simulink model "L400_airframe"  (R2024b)
settings: Solver=FixedStepAuto  StartTime=0  StopTime=10  FixedStep=5/1000  RelTol=1e-3
values from neighbouring files (symbols this model uses):
  db =     [L400_airframe_data.mat]
undefined symbols (not defined in the file or in its folder): lambda
libraries: aerolibconvert2 x16, simulink x6, matrix_library x4, aerolibactuator x2, shared6dof x1, aerolibtransform2 x1
(part 3 of 4)

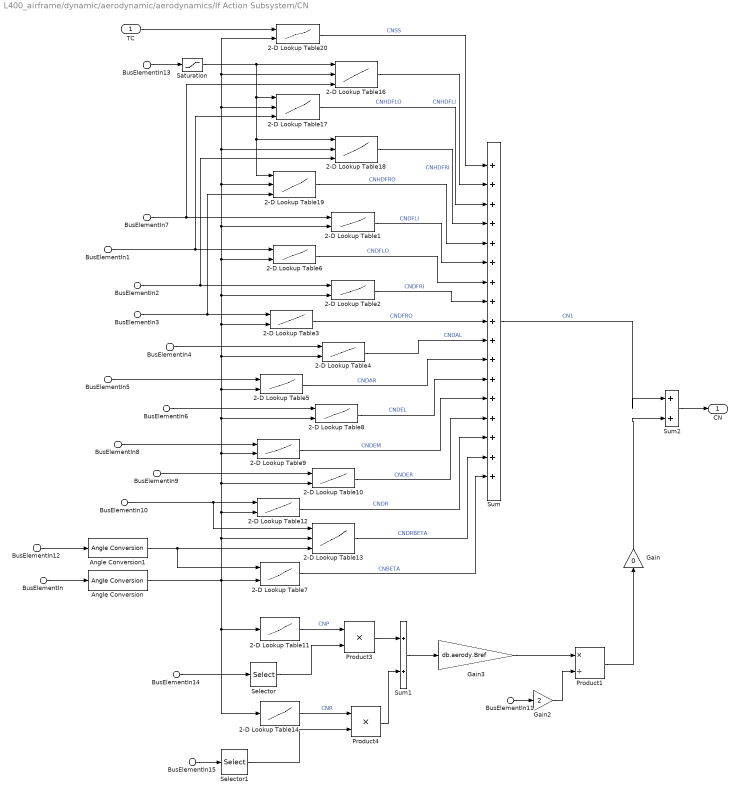
== system L400_airframe/dynamic/aerodynamic/aerodynamics/If Action Subsystem/CN ==
  TC : Inport
  BusElementIn7 : Inport  Port=2  PortName=surface  Element=DFLI
  BusElementIn1 : Inport  Port=2  PortName=surface  Element=DFLO
  BusElementIn2 : Inport  Port=2  PortName=surface  Element=DFRI
  BusElementIn3 : Inport  Port=2  PortName=surface  Element=DFRO
  BusElementIn4 : Inport  Port=2  PortName=surface  Element=DAL
  BusElementIn5 : Inport  Port=2  PortName=surface  Element=DAR
  BusElementIn6 : Inport  Port=2  PortName=surface  Element=DEL
  BusElementIn8 : Inport  Port=2  PortName=surface  Element=DEM
  BusElementIn9 : Inport  Port=2  PortName=surface  Element=DER
  BusElementIn10 : Inport  Port=2  PortName=surface  Element=DR
  BusElementIn : Inport  Port=3  PortName=state  Element=aircraft.airdata.alpha
  BusElementIn12 : Inport  Port=3  PortName=state  Element=aircraft.airdata.beta
  BusElementIn11 : Inport  Port=3  PortName=state  Element=aircraft.airdata.airspeed
  BusElementIn13 : Inport  Port=3  PortName=state  Element=aircraft.position.agl
  BusElementIn14 : Inport  Port=3  PortName=state  Element=aircraft.attitude.p_q_r
  BusElementIn15 : Inport  Port=3  PortName=state  Element=aircraft.attitude.p_q_r
  2-D Lookup Table1 : Lookup_n-D  LookupTableObject=''  BreakpointsForDimension1=db.aerody.VDF  BreakpointsForDimension2=db.aerody.VALPHA  BreakpointsForDimension1FirstPoint=10  BreakpointsForDimension2FirstPoint=10  BreakpointsForDimension1Spacing=12  BreakpointsForDimension2Spacing=12  IndexSearchMethod=Linear search  BeginIndexSearchUsingPreviousIndexResult=on  Table=db.aerody.CNDFLI  ExtrapMethod=Clip  DiagnosticForOutOfRangeInput=Warning  InternalRulePriority=Speed  RndMeth=Simplest
      settings: InputPortMap=u0,u1
  2-D Lookup Table10 : Lookup_n-D  LookupTableObject=''  BreakpointsForDimension1=db.aerody.VDE  BreakpointsForDimension2=db.aerody.VALPHA  BreakpointsForDimension1FirstPoint=10  BreakpointsForDimension2FirstPoint=10  BreakpointsForDimension1Spacing=12  BreakpointsForDimension2Spacing=12  IndexSearchMethod=Linear search  BeginIndexSearchUsingPreviousIndexResult=on  Table=db.aerody.CNDER  ExtrapMethod=Clip  DiagnosticForOutOfRangeInput=Warning  InternalRulePriority=Speed  RndMeth=Simplest
      settings: InputPortMap=u0,u1
  2-D Lookup Table11 : Lookup_n-D  NumberOfTableDimensions=1  LookupTableObject=''  BreakpointsForDimension1=db.dds.VALPHA  BreakpointsForDimension2=db.aerody.VALPHA  BreakpointsForDimension1FirstPoint=10  BreakpointsForDimension2FirstPoint=10  BreakpointsForDimension1Spacing=12  BreakpointsForDimension2Spacing=12  IndexSearchMethod=Linear search  BeginIndexSearchUsingPreviousIndexResult=on  Table=db.dds.CNP  ExtrapMethod=Clip  DiagnosticForOutOfRangeInput=Warning  InternalRulePriority=Speed  RndMeth=Simplest
  2-D Lookup Table12 : Lookup_n-D  LookupTableObject=''  BreakpointsForDimension1=db.aerody.VDR  BreakpointsForDimension2=db.aerody.VALPHA  BreakpointsForDimension1FirstPoint=10  BreakpointsForDimension2FirstPoint=10  BreakpointsForDimension1Spacing=12  BreakpointsForDimension2Spacing=12  IndexSearchMethod=Linear search  BeginIndexSearchUsingPreviousIndexResult=on  Table=db.aerody.CNDR  ExtrapMethod=Clip  DiagnosticForOutOfRangeInput=Warning  InternalRulePriority=Speed  RndMeth=Simplest
      settings: InputPortMap=u0,u1
  2-D Lookup Table13 : Lookup_n-D  NumberOfTableDimensions=3  LookupTableObject=''  BreakpointsForDimension1=db.aerody.VDR  BreakpointsForDimension2=db.aerody.VALPHA  BreakpointsForDimension3=db.aerody.VBETA  BreakpointsForDimension1FirstPoint=10  BreakpointsForDimension2FirstPoint=10  BreakpointsForDimension1Spacing=12  BreakpointsForDimension2Spacing=12  IndexSearchMethod=Linear search  BeginIndexSearchUsingPreviousIndexResult=on  Table=db.aerody.CNDRBETA  ExtrapMethod=Clip  DiagnosticForOutOfRangeInput=Warning  InternalRulePriority=Speed  RndMeth=Simplest
      settings: InputPortMap=u0,u1,u2
  2-D Lookup Table14 : Lookup_n-D  NumberOfTableDimensions=1  LookupTableObject=''  BreakpointsForDimension1=db.dds.VALPHA  BreakpointsForDimension2=db.aerody.VALPHA  BreakpointsForDimension1FirstPoint=10  BreakpointsForDimension2FirstPoint=10  BreakpointsForDimension1Spacing=12  BreakpointsForDimension2Spacing=12  IndexSearchMethod=Linear search  BeginIndexSearchUsingPreviousIndexResult=on  Table=db.dds.CNR  ExtrapMethod=Clip  DiagnosticForOutOfRangeInput=Warning  InternalRulePriority=Speed  RndMeth=Simplest
  2-D Lookup Table16 : Lookup_n-D  NumberOfTableDimensions=3  LookupTableObject=''  BreakpointsForDimension1=db.aerody.VH  BreakpointsForDimension2=db.aerody.VALPHA  BreakpointsForDimension3=db.aerody.VDF  BreakpointsForDimension1FirstPoint=10  BreakpointsForDimension2FirstPoint=10  BreakpointsForDimension1Spacing=12  BreakpointsForDimension2Spacing=12  IndexSearchMethod=Linear search  BeginIndexSearchUsingPreviousIndexResult=on  Table=db.aerody.CNHDFLI  ExtrapMethod=Clip  DiagnosticForOutOfRangeInput=Warning  InternalRulePriority=Speed  RndMeth=Simplest
      settings: InputPortMap=u0,u1,u2
  2-D Lookup Table17 : Lookup_n-D  NumberOfTableDimensions=3  LookupTableObject=''  BreakpointsForDimension1=db.aerody.VH  BreakpointsForDimension2=db.aerody.VALPHA  BreakpointsForDimension3=db.aerody.VDF  BreakpointsForDimension1FirstPoint=10  BreakpointsForDimension2FirstPoint=10  BreakpointsForDimension1Spacing=12  BreakpointsForDimension2Spacing=12  IndexSearchMethod=Linear search  BeginIndexSearchUsingPreviousIndexResult=on  Table=db.aerody.CNHDFLO  ExtrapMethod=Clip  DiagnosticForOutOfRangeInput=Warning  InternalRulePriority=Speed  RndMeth=Simplest
      settings: InputPortMap=u0,u1,u2
  2-D Lookup Table18 : Lookup_n-D  NumberOfTableDimensions=3  LookupTableObject=''  BreakpointsForDimension1=db.aerody.VH  BreakpointsForDimension2=db.aerody.VALPHA  BreakpointsForDimension3=db.aerody.VDF  BreakpointsForDimension1FirstPoint=10  BreakpointsForDimension2FirstPoint=10  BreakpointsForDimension1Spacing=12  BreakpointsForDimension2Spacing=12  IndexSearchMethod=Linear search  BeginIndexSearchUsingPreviousIndexResult=on  Table=db.aerody.CNHDFRI  ExtrapMethod=Clip  DiagnosticForOutOfRangeInput=Warning  InternalRulePriority=Speed  RndMeth=Simplest
      settings: InputPortMap=u0,u1,u2
  2-D Lookup Table19 : Lookup_n-D  NumberOfTableDimensions=3  LookupTableObject=''  BreakpointsForDimension1=db.aerody.VH  BreakpointsForDimension2=db.aerody.VALPHA  BreakpointsForDimension3=db.aerody.VDF  BreakpointsForDimension1FirstPoint=10  BreakpointsForDimension2FirstPoint=10  BreakpointsForDimension1Spacing=12  BreakpointsForDimension2Spacing=12  IndexSearchMethod=Linear search  BeginIndexSearchUsingPreviousIndexResult=on  Table=db.aerody.CNHDFRO  ExtrapMethod=Clip  DiagnosticForOutOfRangeInput=Warning  InternalRulePriority=Speed  RndMeth=Simplest
      settings: InputPortMap=u0,u1,u2
  2-D Lookup Table2 : Lookup_n-D  LookupTableObject=''  BreakpointsForDimension1=db.aerody.VDF  BreakpointsForDimension2=db.aerody.VALPHA  BreakpointsForDimension1FirstPoint=10  BreakpointsForDimension2FirstPoint=10  BreakpointsForDimension1Spacing=12  BreakpointsForDimension2Spacing=12  IndexSearchMethod=Linear search  BeginIndexSearchUsingPreviousIndexResult=on  Table=db.aerody.CNDFRI  ExtrapMethod=Clip  DiagnosticForOutOfRangeInput=Warning  InternalRulePriority=Speed  RndMeth=Simplest
      settings: InputPortMap=u0,u1
  2-D Lookup Table20 : Lookup_n-D  LookupTableObject=''  BreakpointsForDimension1=db.aerody.VTC  BreakpointsForDimension2=db.aerody.VALPHA  BreakpointsForDimension1FirstPoint=10  BreakpointsForDimension2FirstPoint=10  BreakpointsForDimension1Spacing=12  BreakpointsForDimension2Spacing=12  IndexSearchMethod=Linear search  BeginIndexSearchUsingPreviousIndexResult=on  Table=db.aerody.CNSS  ExtrapMethod=Clip  DiagnosticForOutOfRangeInput=Warning  InternalRulePriority=Speed  RndMeth=Simplest
      settings: InputPortMap=u0,u1
  2-D Lookup Table3 : Lookup_n-D  LookupTableObject=''  BreakpointsForDimension1=db.aerody.VDF  BreakpointsForDimension2=db.aerody.VALPHA  BreakpointsForDimension1FirstPoint=10  BreakpointsForDimension2FirstPoint=10  BreakpointsForDimension1Spacing=12  BreakpointsForDimension2Spacing=12  IndexSearchMethod=Linear search  BeginIndexSearchUsingPreviousIndexResult=on  Table=db.aerody.CNDFRO  ExtrapMethod=Clip  DiagnosticForOutOfRangeInput=Warning  InternalRulePriority=Speed  RndMeth=Simplest
      settings: InputPortMap=u0,u1
  2-D Lookup Table4 : Lookup_n-D  LookupTableObject=''  BreakpointsForDimension1=db.aerody.VDA  BreakpointsForDimension2=db.aerody.VALPHA  BreakpointsForDimension1FirstPoint=10  BreakpointsForDimension2FirstPoint=10  BreakpointsForDimension1Spacing=12  BreakpointsForDimension2Spacing=12  IndexSearchMethod=Linear search  BeginIndexSearchUsingPreviousIndexResult=on  Table=db.aerody.CNDAL  ExtrapMethod=Clip  DiagnosticForOutOfRangeInput=Warning  InternalRulePriority=Speed  RndMeth=Simplest
      settings: InputPortMap=u0,u1
  2-D Lookup Table5 : Lookup_n-D  LookupTableObject=''  BreakpointsForDimension1=db.aerody.VDA  BreakpointsForDimension2=db.aerody.VALPHA  BreakpointsForDimension1FirstPoint=10  BreakpointsForDimension2FirstPoint=10  BreakpointsForDimension1Spacing=12  BreakpointsForDimension2Spacing=12  IndexSearchMethod=Linear search  BeginIndexSearchUsingPreviousIndexResult=on  Table=db.aerody.CNDAR  ExtrapMethod=Clip  DiagnosticForOutOfRangeInput=Warning  InternalRulePriority=Speed  RndMeth=Simplest
      settings: InputPortMap=u0,u1
  2-D Lookup Table6 : Lookup_n-D  LookupTableObject=''  BreakpointsForDimension1=db.aerody.VDF  BreakpointsForDimension2=db.aerody.VALPHA  BreakpointsForDimension1FirstPoint=10  BreakpointsForDimension2FirstPoint=10  BreakpointsForDimension1Spacing=12  BreakpointsForDimension2Spacing=12  IndexSearchMethod=Linear search  BeginIndexSearchUsingPreviousIndexResult=on  Table=db.aerody.CNDFLO  ExtrapMethod=Clip  DiagnosticForOutOfRangeInput=Warning  InternalRulePriority=Speed  RndMeth=Simplest
      settings: InputPortMap=u0,u1
  2-D Lookup Table7 : Lookup_n-D  LookupTableObject=''  BreakpointsForDimension1=db.aerody.VBETA  BreakpointsForDimension2=db.aerody.VALPHA  BreakpointsForDimension1FirstPoint=10  BreakpointsForDimension2FirstPoint=10  BreakpointsForDimension1Spacing=12  BreakpointsForDimension2Spacing=12  IndexSearchMethod=Linear search  BeginIndexSearchUsingPreviousIndexResult=on  Table=db.aerody.CNBETA  ExtrapMethod=Clip  DiagnosticForOutOfRangeInput=Warning  InternalRulePriority=Speed  RndMeth=Simplest
      settings: InputPortMap=u0,u1
  2-D Lookup Table8 : Lookup_n-D  LookupTableObject=''  BreakpointsForDimension1=db.aerody.VDE  BreakpointsForDimension2=db.aerody.VALPHA  BreakpointsForDimension1FirstPoint=10  BreakpointsForDimension2FirstPoint=10  BreakpointsForDimension1Spacing=12  BreakpointsForDimension2Spacing=12  IndexSearchMethod=Linear search  BeginIndexSearchUsingPreviousIndexResult=on  Table=db.aerody.CNDEL  ExtrapMethod=Clip  DiagnosticForOutOfRangeInput=Warning  InternalRulePriority=Speed  RndMeth=Simplest
      settings: InputPortMap=u0,u1
  2-D Lookup Table9 : Lookup_n-D  LookupTableObject=''  BreakpointsForDimension1=db.aerody.VDE  BreakpointsForDimension2=db.aerody.VALPHA  BreakpointsForDimension1FirstPoint=10  BreakpointsForDimension2FirstPoint=10  BreakpointsForDimension1Spacing=12  BreakpointsForDimension2Spacing=12  IndexSearchMethod=Linear search  BeginIndexSearchUsingPreviousIndexResult=on  Table=db.aerody.CNDEM  ExtrapMethod=Clip  DiagnosticForOutOfRangeInput=Warning  InternalRulePriority=Speed  RndMeth=Simplest
      settings: InputPortMap=u0,u1
  Angle Conversion : aerolibconvert2/Angle Conversion  IU=rad  OU=deg
  Angle Conversion1 : aerolibconvert2/Angle Conversion  IU=rad  OU=deg
  Gain : Gain  Gain=0
  Gain2 : Gain  Gain=2
  Gain3 : Gain  Gain=db.aerody.Bref
  Product1 : Product  Inputs=*/
  Product3 : Product  Inputs=**
  Product4 : Product  Inputs=**
  Saturation : Saturate  UpperLimit=5.8  LowerLimit=0
  Selector : Selector  InputPortWidth=3  IndexOptions=Index vector (dialog)  Indices=1  OutputSizes=1
  Selector1 : Selector  InputPortWidth=3  IndexOptions=Index vector (dialog)  Indices=3  OutputSizes=1
  Sum : Sum  Inputs=17
  Sum1 : Sum  Inputs=2
  Sum2 : Sum  Inputs=|++
  CN : Outport
  wires:
  BusElementIn12/1 -> Angle Conversion1/1
  Sum/1 -> Sum2/1  "CN1"
  BusElementIn7/1 -> 2-D Lookup Table16/3, 2-D Lookup Table1/1
  BusElementIn1/1 -> 2-D Lookup Table17/3, 2-D Lookup Table6/1
  BusElementIn2/1 -> 2-D Lookup Table18/3, 2-D Lookup Table2/1
  BusElementIn3/1 -> 2-D Lookup Table19/3, 2-D Lookup Table3/1
  BusElementIn4/1 -> 2-D Lookup Table4/1
  BusElementIn5/1 -> 2-D Lookup Table5/1
  BusElementIn6/1 -> 2-D Lookup Table8/1
  BusElementIn8/1 -> 2-D Lookup Table9/1
  BusElementIn9/1 -> 2-D Lookup Table10/1
  BusElementIn10/1 -> 2-D Lookup Table13/1, 2-D Lookup Table12/1
  BusElementIn13/1 -> Saturation/1
  TC/1 -> 2-D Lookup Table20/1
  BusElementIn/1 -> Angle Conversion/1
  2-D Lookup Table2/1 -> Sum/8  "CNDFRI"
  2-D Lookup Table4/1 -> Sum/10  "CNDAL"
  2-D Lookup Table1/1 -> Sum/6  "CNDFLI"
  2-D Lookup Table3/1 -> Sum/9  "CNDFRO"
  2-D Lookup Table8/1 -> Sum/12  "CNDEL"
  2-D Lookup Table18/1 -> Sum/4  "CNHDFRI"
  2-D Lookup Table6/1 -> Sum/7  "CNDFLO"
  2-D Lookup Table5/1 -> Sum/11  "CNDAR"
  2-D Lookup Table10/1 -> Sum/14  "CNDER"
  2-D Lookup Table16/1 -> Sum/2  "CNHDFLI"
  2-D Lookup Table19/1 -> Sum/5  "CNHDFRO"
  2-D Lookup Table9/1 -> Sum/13  "CNDEM"
  2-D Lookup Table13/1 -> Sum/16  "CNDRBETA"
  2-D Lookup Table17/1 -> Sum/3  "CNHDFLO"
  2-D Lookup Table12/1 -> Sum/15  "CNDR"
  2-D Lookup Table20/1 -> Sum/1  "CNSS"
  2-D Lookup Table7/1 -> Sum/17  "CNBETA"
  Sum1/1 -> Gain3/1
  BusElementIn11/1 -> Gain2/1
  Selector1/1 -> Product4/2
  Selector/1 -> Product3/2
  2-D Lookup Table11/1 -> Product3/1  "CNP"
  2-D Lookup Table14/1 -> Product4/1  "CNR"
  Product3/1 -> Sum1/1
  Product4/1 -> Sum1/2
  Product1/1 -> Gain/1
  Sum2/1 -> CN/1
  Angle Conversion/1 -> 2-D Lookup Table14/1, 2-D Lookup Table11/1, 2-D Lookup Table20/2, 2-D Lookup Table16/2, 2-D Lookup Table17/2, 2-D Lookup Table18/2, 2-D Lookup Table19/2, 2-D Lookup Table1/2, 2-D Lookup Table6/2, 2-D Lookup Table2/2, 2-D Lookup Table3/2, 2-D Lookup Table4/2, 2-D Lookup Table5/2, 2-D Lookup Table8/2, 2-D Lookup Table9/2, 2-D Lookup Table10/2, 2-D Lookup Table12/2, 2-D Lookup Table13/2, 2-D Lookup Table7/2
  Angle Conversion1/1 -> 2-D Lookup Table7/1, 2-D Lookup Table13/3
  BusElementIn15/1 -> Selector1/1
  BusElementIn14/1 -> Selector/1
  Saturation/1 -> 2-D Lookup Table17/1, 2-D Lookup Table18/1, 2-D Lookup Table19/1, 2-D Lookup Table16/1
  Gain3/1 -> Product1/1
  Gain2/1 -> Product1/2
  Gain/1 -> Sum2/2

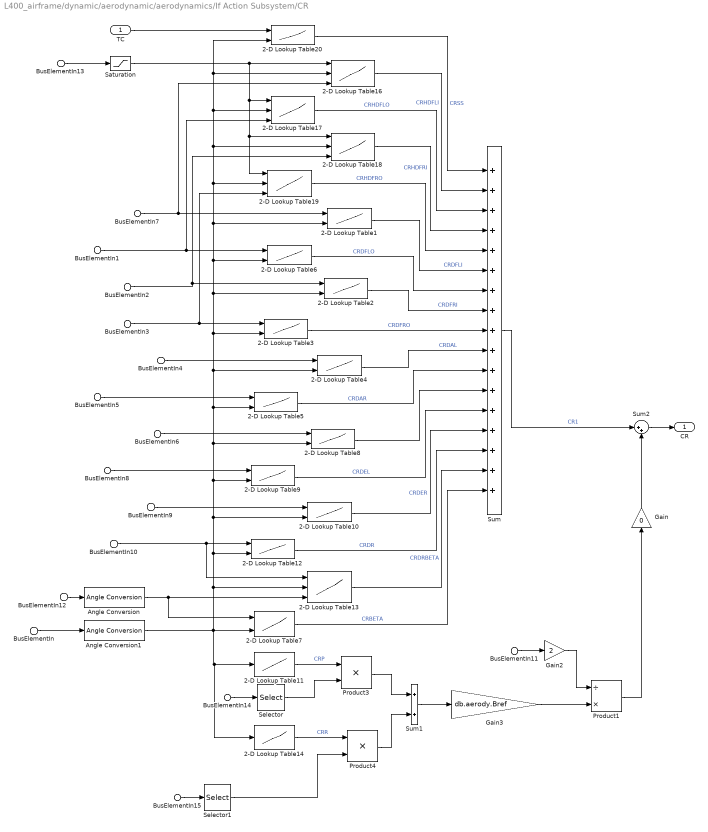
== system L400_airframe/dynamic/aerodynamic/aerodynamics/If Action Subsystem/CR ==
  TC : Inport
  BusElementIn7 : Inport  Port=2  PortName=surface  Element=DFLI
  BusElementIn1 : Inport  Port=2  PortName=surface  Element=DFLO
  BusElementIn2 : Inport  Port=2  PortName=surface  Element=DFRI
  BusElementIn3 : Inport  Port=2  PortName=surface  Element=DFRO
  BusElementIn4 : Inport  Port=2  PortName=surface  Element=DAL
  BusElementIn5 : Inport  Port=2  PortName=surface  Element=DAR
  BusElementIn6 : Inport  Port=2  PortName=surface  Element=DEL
  BusElementIn8 : Inport  Port=2  PortName=surface  Element=DEM
  BusElementIn9 : Inport  Port=2  PortName=surface  Element=DER
  BusElementIn10 : Inport  Port=2  PortName=surface  Element=DR
  BusElementIn : Inport  Port=3  PortName=state  Element=aircraft.airdata.alpha
  BusElementIn12 : Inport  Port=3  PortName=state  Element=aircraft.airdata.beta
  BusElementIn11 : Inport  Port=3  PortName=state  Element=aircraft.airdata.airspeed
  BusElementIn13 : Inport  Port=3  PortName=state  Element=aircraft.position.agl
  BusElementIn14 : Inport  Port=3  PortName=state  Element=aircraft.attitude.p_q_r
  BusElementIn15 : Inport  Port=3  PortName=state  Element=aircraft.attitude.p_q_r
  2-D Lookup Table1 : Lookup_n-D  LookupTableObject=''  BreakpointsForDimension1=db.aerody.VDF  BreakpointsForDimension2=db.aerody.VALPHA  BreakpointsForDimension1FirstPoint=10  BreakpointsForDimension2FirstPoint=10  BreakpointsForDimension1Spacing=12  BreakpointsForDimension2Spacing=12  IndexSearchMethod=Linear search  BeginIndexSearchUsingPreviousIndexResult=on  Table=db.aerody.CRDFLI  ExtrapMethod=Clip  DiagnosticForOutOfRangeInput=Warning  InternalRulePriority=Speed  RndMeth=Simplest
      settings: InputPortMap=u0,u1
  2-D Lookup Table10 : Lookup_n-D  LookupTableObject=''  BreakpointsForDimension1=db.aerody.VDE  BreakpointsForDimension2=db.aerody.VALPHA  BreakpointsForDimension1FirstPoint=10  BreakpointsForDimension2FirstPoint=10  BreakpointsForDimension1Spacing=12  BreakpointsForDimension2Spacing=12  IndexSearchMethod=Linear search  BeginIndexSearchUsingPreviousIndexResult=on  Table=db.aerody.CRDER  ExtrapMethod=Clip  DiagnosticForOutOfRangeInput=Warning  InternalRulePriority=Speed  RndMeth=Simplest
      settings: InputPortMap=u0,u1
  2-D Lookup Table11 : Lookup_n-D  NumberOfTableDimensions=1  LookupTableObject=''  BreakpointsForDimension1=db.dds.VALPHA  BreakpointsForDimension2=db.aerody.VALPHA  BreakpointsForDimension1FirstPoint=10  BreakpointsForDimension2FirstPoint=10  BreakpointsForDimension1Spacing=12  BreakpointsForDimension2Spacing=12  IndexSearchMethod=Linear search  BeginIndexSearchUsingPreviousIndexResult=on  Table=db.dds.CRP  ExtrapMethod=Clip  DiagnosticForOutOfRangeInput=Warning  InternalRulePriority=Speed  RndMeth=Simplest
  2-D Lookup Table12 : Lookup_n-D  LookupTableObject=''  BreakpointsForDimension1=db.aerody.VDR  BreakpointsForDimension2=db.aerody.VALPHA  BreakpointsForDimension1FirstPoint=10  BreakpointsForDimension2FirstPoint=10  BreakpointsForDimension1Spacing=12  BreakpointsForDimension2Spacing=12  IndexSearchMethod=Linear search  BeginIndexSearchUsingPreviousIndexResult=on  Table=db.aerody.CRDR  ExtrapMethod=Clip  DiagnosticForOutOfRangeInput=Warning  InternalRulePriority=Speed  RndMeth=Simplest
      settings: InputPortMap=u0,u1
  2-D Lookup Table13 : Lookup_n-D  NumberOfTableDimensions=3  LookupTableObject=''  BreakpointsForDimension1=db.aerody.VDR  BreakpointsForDimension2=db.aerody.VALPHA  BreakpointsForDimension3=db.aerody.VBETA  BreakpointsForDimension1FirstPoint=10  BreakpointsForDimension2FirstPoint=10  BreakpointsForDimension1Spacing=12  BreakpointsForDimension2Spacing=12  IndexSearchMethod=Linear search  BeginIndexSearchUsingPreviousIndexResult=on  Table=db.aerody.CRDRBETA  ExtrapMethod=Clip  DiagnosticForOutOfRangeInput=Warning  InternalRulePriority=Speed  RndMeth=Simplest
      settings: InputPortMap=u0,u1,u2
  2-D Lookup Table14 : Lookup_n-D  NumberOfTableDimensions=1  LookupTableObject=''  BreakpointsForDimension1=db.dds.VALPHA  BreakpointsForDimension2=db.aerody.VALPHA  BreakpointsForDimension1FirstPoint=10  BreakpointsForDimension2FirstPoint=10  BreakpointsForDimension1Spacing=12  BreakpointsForDimension2Spacing=12  IndexSearchMethod=Linear search  BeginIndexSearchUsingPreviousIndexResult=on  Table=db.dds.CRR  ExtrapMethod=Clip  DiagnosticForOutOfRangeInput=Warning  InternalRulePriority=Speed  RndMeth=Simplest
  2-D Lookup Table16 : Lookup_n-D  NumberOfTableDimensions=3  LookupTableObject=''  BreakpointsForDimension1=db.aerody.VH  BreakpointsForDimension2=db.aerody.VALPHA  BreakpointsForDimension3=db.aerody.VDF  BreakpointsForDimension1FirstPoint=10  BreakpointsForDimension2FirstPoint=10  BreakpointsForDimension1Spacing=12  BreakpointsForDimension2Spacing=12  IndexSearchMethod=Linear search  BeginIndexSearchUsingPreviousIndexResult=on  Table=db.aerody.CRHDFLI  ExtrapMethod=Clip  DiagnosticForOutOfRangeInput=Warning  InternalRulePriority=Speed  RndMeth=Simplest
      settings: InputPortMap=u0,u1,u2
  2-D Lookup Table17 : Lookup_n-D  NumberOfTableDimensions=3  LookupTableObject=''  BreakpointsForDimension1=db.aerody.VH  BreakpointsForDimension2=db.aerody.VALPHA  BreakpointsForDimension3=db.aerody.VDF  BreakpointsForDimension1FirstPoint=10  BreakpointsForDimension2FirstPoint=10  BreakpointsForDimension1Spacing=12  BreakpointsForDimension2Spacing=12  IndexSearchMethod=Linear search  BeginIndexSearchUsingPreviousIndexResult=on  Table=db.aerody.CRHDFLO  ExtrapMethod=Clip  DiagnosticForOutOfRangeInput=Warning  InternalRulePriority=Speed  RndMeth=Simplest
      settings: InputPortMap=u0,u1,u2
  2-D Lookup Table18 : Lookup_n-D  NumberOfTableDimensions=3  LookupTableObject=''  BreakpointsForDimension1=db.aerody.VH  BreakpointsForDimension2=db.aerody.VALPHA  BreakpointsForDimension3=db.aerody.VDF  BreakpointsForDimension1FirstPoint=10  BreakpointsForDimension2FirstPoint=10  BreakpointsForDimension1Spacing=12  BreakpointsForDimension2Spacing=12  IndexSearchMethod=Linear search  BeginIndexSearchUsingPreviousIndexResult=on  Table=db.aerody.CRHDFRI  ExtrapMethod=Clip  DiagnosticForOutOfRangeInput=Warning  InternalRulePriority=Speed  RndMeth=Simplest
      settings: InputPortMap=u0,u1,u2
  2-D Lookup Table19 : Lookup_n-D  NumberOfTableDimensions=3  LookupTableObject=''  BreakpointsForDimension1=db.aerody.VH  BreakpointsForDimension2=db.aerody.VALPHA  BreakpointsForDimension3=db.aerody.VDF  BreakpointsForDimension1FirstPoint=10  BreakpointsForDimension2FirstPoint=10  BreakpointsForDimension1Spacing=12  BreakpointsForDimension2Spacing=12  IndexSearchMethod=Linear search  BeginIndexSearchUsingPreviousIndexResult=on  Table=db.aerody.CRHDFRO  ExtrapMethod=Clip  DiagnosticForOutOfRangeInput=Warning  InternalRulePriority=Speed  RndMeth=Simplest
      settings: InputPortMap=u0,u1,u2
  2-D Lookup Table2 : Lookup_n-D  LookupTableObject=''  BreakpointsForDimension1=db.aerody.VDF  BreakpointsForDimension2=db.aerody.VALPHA  BreakpointsForDimension1FirstPoint=10  BreakpointsForDimension2FirstPoint=10  BreakpointsForDimension1Spacing=12  BreakpointsForDimension2Spacing=12  IndexSearchMethod=Linear search  BeginIndexSearchUsingPreviousIndexResult=on  Table=db.aerody.CRDFRI  ExtrapMethod=Clip  DiagnosticForOutOfRangeInput=Warning  InternalRulePriority=Speed  RndMeth=Simplest
      settings: InputPortMap=u0,u1
  2-D Lookup Table20 : Lookup_n-D  LookupTableObject=''  BreakpointsForDimension1=db.aerody.VTC  BreakpointsForDimension2=db.aerody.VALPHA  BreakpointsForDimension1FirstPoint=10  BreakpointsForDimension2FirstPoint=10  BreakpointsForDimension1Spacing=12  BreakpointsForDimension2Spacing=12  IndexSearchMethod=Linear search  BeginIndexSearchUsingPreviousIndexResult=on  Table=db.aerody.CRSS  ExtrapMethod=Clip  DiagnosticForOutOfRangeInput=Warning  InternalRulePriority=Speed  RndMeth=Simplest
      settings: InputPortMap=u0,u1
  2-D Lookup Table3 : Lookup_n-D  LookupTableObject=''  BreakpointsForDimension1=db.aerody.VDF  BreakpointsForDimension2=db.aerody.VALPHA  BreakpointsForDimension1FirstPoint=10  BreakpointsForDimension2FirstPoint=10  BreakpointsForDimension1Spacing=12  BreakpointsForDimension2Spacing=12  IndexSearchMethod=Linear search  BeginIndexSearchUsingPreviousIndexResult=on  Table=db.aerody.CRDFRO  ExtrapMethod=Clip  DiagnosticForOutOfRangeInput=Warning  InternalRulePriority=Speed  RndMeth=Simplest
      settings: InputPortMap=u0,u1
  2-D Lookup Table4 : Lookup_n-D  LookupTableObject=''  BreakpointsForDimension1=db.aerody.VDA  BreakpointsForDimension2=db.aerody.VALPHA  BreakpointsForDimension1FirstPoint=10  BreakpointsForDimension2FirstPoint=10  BreakpointsForDimension1Spacing=12  BreakpointsForDimension2Spacing=12  IndexSearchMethod=Linear search  BeginIndexSearchUsingPreviousIndexResult=on  Table=db.aerody.CRDAL  ExtrapMethod=Clip  DiagnosticForOutOfRangeInput=Warning  InternalRulePriority=Speed  RndMeth=Simplest
      settings: InputPortMap=u0,u1
  2-D Lookup Table5 : Lookup_n-D  LookupTableObject=''  BreakpointsForDimension1=db.aerody.VDA  BreakpointsForDimension2=db.aerody.VALPHA  BreakpointsForDimension1FirstPoint=10  BreakpointsForDimension2FirstPoint=10  BreakpointsForDimension1Spacing=12  BreakpointsForDimension2Spacing=12  IndexSearchMethod=Linear search  BeginIndexSearchUsingPreviousIndexResult=on  Table=db.aerody.CRDAR  ExtrapMethod=Clip  DiagnosticForOutOfRangeInput=Warning  InternalRulePriority=Speed  RndMeth=Simplest
      settings: InputPortMap=u0,u1
  2-D Lookup Table6 : Lookup_n-D  LookupTableObject=''  BreakpointsForDimension1=db.aerody.VDF  BreakpointsForDimension2=db.aerody.VALPHA  BreakpointsForDimension1FirstPoint=10  BreakpointsForDimension2FirstPoint=10  BreakpointsForDimension1Spacing=12  BreakpointsForDimension2Spacing=12  IndexSearchMethod=Linear search  BeginIndexSearchUsingPreviousIndexResult=on  Table=db.aerody.CRDFLO  ExtrapMethod=Clip  DiagnosticForOutOfRangeInput=Warning  InternalRulePriority=Speed  RndMeth=Simplest
      settings: InputPortMap=u0,u1
  2-D Lookup Table7 : Lookup_n-D  LookupTableObject=''  BreakpointsForDimension1=db.aerody.VBETA  BreakpointsForDimension2=db.aerody.VALPHA  BreakpointsForDimension1FirstPoint=10  BreakpointsForDimension2FirstPoint=10  BreakpointsForDimension1Spacing=12  BreakpointsForDimension2Spacing=12  IndexSearchMethod=Linear search  BeginIndexSearchUsingPreviousIndexResult=on  Table=db.aerody.CRBETA  ExtrapMethod=Clip  DiagnosticForOutOfRangeInput=Warning  InternalRulePriority=Speed  RndMeth=Simplest
      settings: InputPortMap=u0,u1
  2-D Lookup Table8 : Lookup_n-D  LookupTableObject=''  BreakpointsForDimension1=db.aerody.VDE  BreakpointsForDimension2=db.aerody.VALPHA  BreakpointsForDimension1FirstPoint=10  BreakpointsForDimension2FirstPoint=10  BreakpointsForDimension1Spacing=12  BreakpointsForDimension2Spacing=12  IndexSearchMethod=Linear search  BeginIndexSearchUsingPreviousIndexResult=on  Table=db.aerody.CRDEL  ExtrapMethod=Clip  DiagnosticForOutOfRangeInput=Warning  InternalRulePriority=Speed  RndMeth=Simplest
      settings: InputPortMap=u0,u1
  2-D Lookup Table9 : Lookup_n-D  LookupTableObject=''  BreakpointsForDimension1=db.aerody.VDE  BreakpointsForDimension2=db.aerody.VALPHA  BreakpointsForDimension1FirstPoint=10  BreakpointsForDimension2FirstPoint=10  BreakpointsForDimension1Spacing=12  BreakpointsForDimension2Spacing=12  IndexSearchMethod=Linear search  BeginIndexSearchUsingPreviousIndexResult=on  Table=db.aerody.CRDEM  ExtrapMethod=Clip  DiagnosticForOutOfRangeInput=Warning  InternalRulePriority=Speed  RndMeth=Simplest
      settings: InputPortMap=u0,u1
  Angle Conversion : aerolibconvert2/Angle Conversion  IU=rad  OU=deg
  Angle Conversion1 : aerolibconvert2/Angle Conversion  IU=rad  OU=deg
  Gain : Gain  Gain=0
  Gain2 : Gain  Gain=2
  Gain3 : Gain  Gain=db.aerody.Bref
  Product1 : Product  Inputs=/*
  Product3 : Product  Inputs=**
  Product4 : Product  Inputs=**
  Saturation : Saturate  UpperLimit=5.8  LowerLimit=0
  Selector : Selector  InputPortWidth=3  IndexOptions=Index vector (dialog)  Indices=1  OutputSizes=1
  Selector1 : Selector  InputPortWidth=3  IndexOptions=Index vector (dialog)  Indices=3  OutputSizes=1
  Sum : Sum  Inputs=17
  Sum1 : Sum  Inputs=2
  Sum2 : Sum  Inputs=|++
  CR : Outport
  wires:
  BusElementIn/1 -> Angle Conversion1/1
  TC/1 -> 2-D Lookup Table20/1
  BusElementIn13/1 -> Saturation/1
  BusElementIn10/1 -> 2-D Lookup Table13/1, 2-D Lookup Table12/1
  BusElementIn9/1 -> 2-D Lookup Table10/1
  BusElementIn8/1 -> 2-D Lookup Table9/1
  BusElementIn6/1 -> 2-D Lookup Table8/1
  BusElementIn5/1 -> 2-D Lookup Table5/1
  BusElementIn4/1 -> 2-D Lookup Table4/1
  BusElementIn3/1 -> 2-D Lookup Table19/3, 2-D Lookup Table3/1
  BusElementIn2/1 -> 2-D Lookup Table18/3, 2-D Lookup Table2/1
  BusElementIn1/1 -> 2-D Lookup Table6/1, 2-D Lookup Table17/3
  BusElementIn7/1 -> 2-D Lookup Table1/1, 2-D Lookup Table16/3
  Sum/1 -> Sum2/1  "CR1"
  BusElementIn12/1 -> Angle Conversion/1
  2-D Lookup Table2/1 -> Sum/8  "CRDFRI"
  2-D Lookup Table1/1 -> Sum/6  "CRDFLI"
  2-D Lookup Table4/1 -> Sum/10  "CRDAL"
  2-D Lookup Table18/1 -> Sum/4  "CRHDFRI"
  2-D Lookup Table6/1 -> Sum/7  "CRDFLO"
  2-D Lookup Table3/1 -> Sum/9  "CRDFRO"
  2-D Lookup Table8/1 -> Sum/12
  2-D Lookup Table16/1 -> Sum/2  "CRHDFLI"
  2-D Lookup Table19/1 -> Sum/5  "CRHDFRO"
  2-D Lookup Table10/1 -> Sum/14  "CRDER"
  2-D Lookup Table5/1 -> Sum/11  "CRDAR"
  2-D Lookup Table17/1 -> Sum/3  "CRHDFLO"
  2-D Lookup Table13/1 -> Sum/16  "CRDRBETA"
  2-D Lookup Table9/1 -> Sum/13  "CRDEL"
  2-D Lookup Table20/1 -> Sum/1  "CRSS"
  2-D Lookup Table12/1 -> Sum/15  "CRDR"
  2-D Lookup Table7/1 -> Sum/17  "CRBETA"
  BusElementIn11/1 -> Gain2/1
  Gain2/1 -> Product1/1
  Gain3/1 -> Product1/2
  Sum1/1 -> Gain3/1
  2-D Lookup Table11/1 -> Product3/1  "CRP"
  2-D Lookup Table14/1 -> Product4/1  "CRR"
  Selector1/1 -> Product4/2
  Selector/1 -> Product3/2
  Product3/1 -> Sum1/1
  Product4/1 -> Sum1/2
  Product1/1 -> Gain/1
  Sum2/1 -> CR/1
  Angle Conversion/1 -> 2-D Lookup Table7/1, 2-D Lookup Table13/3
  Angle Conversion1/1 -> 2-D Lookup Table14/1, 2-D Lookup Table11/1, 2-D Lookup Table20/2, 2-D Lookup Table16/2, 2-D Lookup Table17/2, 2-D Lookup Table18/2, 2-D Lookup Table19/2, 2-D Lookup Table1/2, 2-D Lookup Table6/2, 2-D Lookup Table2/2, 2-D Lookup Table3/2, 2-D Lookup Table4/2, 2-D Lookup Table5/2, 2-D Lookup Table8/2, 2-D Lookup Table9/2, 2-D Lookup Table10/2, 2-D Lookup Table12/2, 2-D Lookup Table13/2, 2-D Lookup Table7/2
  BusElementIn14/1 -> Selector/1
  BusElementIn15/1 -> Selector1/1
  Saturation/1 -> 2-D Lookup Table19/1, 2-D Lookup Table18/1, 2-D Lookup Table17/1, 2-D Lookup Table16/1
  Gain/1 -> Sum2/2

== system L400_airframe/dynamic/aerodynamic/aerodynamics/If Action Subsystem/CY ==
  TC : Inport
  BusElementIn7 : Inport  Port=2  PortName=surface  Element=DFLI
  BusElementIn1 : Inport  Port=2  PortName=surface  Element=DFLO
  BusElementIn2 : Inport  Port=2  PortName=surface  Element=DFRI
  BusElementIn3 : Inport  Port=2  PortName=surface  Element=DFRO
  BusElementIn4 : Inport  Port=2  PortName=surface  Element=DAL
  BusElementIn5 : Inport  Port=2  PortName=surface  Element=DAR
  BusElementIn6 : Inport  Port=2  PortName=surface  Element=DEL
  BusElementIn8 : Inport  Port=2  PortName=surface  Element=DEM
  BusElementIn9 : Inport  Port=2  PortName=surface  Element=DER
  BusElementIn10 : Inport  Port=2  PortName=surface  Element=DR
  BusElementIn : Inport  Port=3  PortName=state  Element=aircraft.airdata.alpha
  BusElementIn12 : Inport  Port=3  PortName=state  Element=aircraft.airdata.beta
  BusElementIn13 : Inport  Port=3  PortName=state  Element=aircraft.position.agl
  Angle Conversion : aerolibconvert2/Angle Conversion  IU=rad  OU=deg
  Angle Conversion1 : aerolibconvert2/Angle Conversion  IU=rad  OU=deg
  Subsystem : Subsystem
  CY : Outport
  wires:
  TC/1 -> Subsystem/4(TC)
  BusElementIn13/1 -> Subsystem/3(H)
  BusElementIn7/1 -> Subsystem/5(DFLI)
  BusElementIn1/1 -> Subsystem/6(DFLO)
  BusElementIn2/1 -> Subsystem/7(DFRI)
  BusElementIn3/1 -> Subsystem/8(DFRO)
  BusElementIn4/1 -> Subsystem/9(DAL)
  BusElementIn5/1 -> Subsystem/10(DAR)
  BusElementIn6/1 -> Subsystem/11(DEL)
  BusElementIn8/1 -> Subsystem/12(DEM)
  BusElementIn9/1 -> Subsystem/13(DER)
  BusElementIn10/1 -> Subsystem/14(DR)
  BusElementIn12/1 -> Angle Conversion1/1
  BusElementIn/1 -> Angle Conversion/1
  Subsystem/1(CY) -> CY/1
  Angle Conversion/1 -> Subsystem/1(alpha)
  Angle Conversion1/1 -> Subsystem/2(beta)

== system L400_airframe/dynamic/aerodynamic/aerodynamics/If Action Subsystem/Subsystem ==
  note: CD和CL转到机体坐标系，CY就在机体坐标系
  CD_CY_CL : Inport
  BusElementIn4 : Inport  Port=2  PortName=state  Element=aircraft.airdata.qbar
  BusElementIn1 : Inport  Port=2  PortName=state  Element=aircraft.airdata.qbar
  BusElementIn : Inport  Port=2  PortName=state  Element=aircraft.airdata.alpha
  CR_CM_CN : Inport  Port=3
  Constant : Constant  Value=db.aerody.COP
  Constant1 : Constant  Value=0
  Direction Cosine Matrix Body to Wind : aerolibtransform2/Direction Cosine Matrix Body to Wind
  Gain : Gain  Gain=db.aerody.Sref
  Gain1 : Gain  Gain=db.aerody.Lref*db.aerody.Sref
  Mux : Mux  Inputs=2
  Product : Product
  Product1 : Product
  Product2 : Product  Multiplication=Matrix(*)
  Transpose : Math  Operator=transpose
  Bus Element Out : Outport  PortName=aerody  Element=Fxyz
  Bus Element Out1 : Outport  PortName=aerody  Element=Mxyz
  Bus Element Out3 : Outport  PortName=aerody  Element=Pxyz
  wires:
  Gain1/1 -> Bus Element Out1/1
  Gain/1 -> Bus Element Out/1
  Transpose/1 -> Product2/1
  Constant/1 -> Bus Element Out3/1
  Direction Cosine Matrix Body to Wind/1 -> Transpose/1
  Product2/1 -> Product/2
  CD_CY_CL/1 -> Product2/2
  Mux/1 -> Direction Cosine Matrix Body to Wind/1
  BusElementIn1/1 -> Product/1
  CR_CM_CN/1 -> Product1/1
  Constant1/1 -> Mux/2
  BusElementIn4/1 -> Product1/2
  BusElementIn/1 -> Mux/1
  Product/1 -> Gain/1
  Product1/1 -> Gain1/1

== system L400_airframe/dynamic/landgear/Simple/left/侧向摩擦力 ==
  note: % Compute the sideforce coefficients using Pacejka's Magic Formula.
      | %
      | % y(x) = D sin {C arctan [Bx - E(Bx - arctan Bx)]}
      | %
      | % Where: B = Stiffness Factor (0.06, here)
      | % C = Shape Factor (2.8, here)
      | % D = Peak Factor (0.8, here)
      | % E = Curvature Factor (1.03, here)
  Bus Element In3 : Inport  PortName=gear  Element=speed
  Bus Element In2 : Inport  PortName=gear  Element=istatic
  Bus Element In1 : Inport  PortName=gear  Element=reaction
  |Fz| : Inport  Port=2
  Angle Conversion : aerolibconvert2/Angle Conversion  IU=rad  OU=deg
  Atan : Trigonometry  Operator=atan
  Atan1 : Trigonometry  Operator=atan
  Atan2 : Trigonometry  Operator=atan2
  Atan3 : Trigonometry
  Demux : Demux  Outputs=2
  Gain : Gain  Gain=0.06
  Gain1 : Gain  Gain=1.03
  Gain2 : Gain  Gain=2.8
  Gain3 : Gain  Gain=0.8
  Product : Product
  Selector1 : Selector  InputPortWidth=3  IndexOptions=Index vector (dialog)  Indices=[2, 1]  OutputSizes=1
  Selector2 : Selector  InputPortWidth=2  IndexOptions=Index vector (dialog)  Indices=2  OutputSizes=1
  Selector3 : Selector  InputPortWidth=3  IndexOptions=Index vector (dialog)  Indices=2  OutputSizes=1
  Sum : Sum  Inputs=+-|
  Sum1 : Sum  Inputs=|+-
  Switch : Switch  Criteria=u2 > Threshold  Threshold=0.5  SaturateOnIntegerOverflow=off  InputSameDT=off
  Unary Minus : UnaryMinus
  Fy : Outport
  wires:
  Unary Minus/1 -> Switch/3
  |Fz|/1 -> Product/2
  Gain3/1 -> Product/1
  Angle Conversion/1 -> Gain/1
  Atan3/1 -> Gain3/1
  Atan2/1 -> Angle Conversion/1
  Gain1/1 -> Sum1/2
  Atan1/1 -> Gain2/1
  Sum/1 -> Gain1/1
  Sum1/1 -> Atan1/1
  Gain2/1 -> Atan3/1
  Atan/1 -> Sum/2
  Gain/1 -> Atan/1, Sum1/1, Sum/1
  Product/1 -> Unary Minus/1
  Selector3/1 -> Switch/1
  Bus Element In1/1 -> Selector3/1
  Bus Element In2/1 -> Selector2/1
  Selector2/1 -> Switch/2
  Demux/1 -> Atan2/1
  Selector1/1 -> Demux/1
  Demux/2 -> Atan2/2
  Bus Element In3/1 -> Selector1/1
  Switch/1 -> Fy/1

== system L400_airframe/dynamic/landgear/Simple/left/地面支反力 ==
  note: 弹簧力刚度系数可以大概如下估算：
      | 无人机重力8000N，一共3个轮胎，假设平衡时轮胎压缩1cm，那么
      | K = 8000/3/0.01 ≈ 2.5e5
      | 弹簧系数一定不要打了，否则很容易发散
  note: 轮胎支反力
  note: 摩擦力
  note: 弹簧力
  note: 起落架缓冲器所提供的缓冲力是起落架提供给飞机支反力的主要组成部分，主要由随压缩行程变化的弹簧力、随压缩速率变化的阻尼力以及缓冲器内部有相对运动而产生的滑动摩擦力组成。
  note: 阻尼力
  Bus Element In1 : Inport  PortName=gear  Element=cmprs
  Bus Element In2 : Inport  PortName=gear  Element=speed
  Gain2 : Gain  Gain=1e5
  Gain3 : Gain  Gain=-1e3
  Gain7 : Gain  Gain=0
  Saturation : Saturate  UpperLimit=0  LowerLimit=-1
  Selector3 : Selector  InputPortWidth=3  IndexOptions=Index vector (dialog)  Indices=3  OutputSizes=1
  Sign : Signum
  Sum3 : Sum  Inputs=3
  Fz : Outport
  wires:
  Bus Element In1/1 -> Saturation/1
  Gain2/1 -> Sum3/1
  Gain3/1 -> Sum3/2
  Selector3/1 -> Gain3/1, Sign/1
  Saturation/1 -> Gain2/1
  Sign/1 -> Gain7/1
  Sum3/1 -> Fz/1
  Bus Element In2/1 -> Selector3/1
  Gain7/1 -> Sum3/3

== system L400_airframe/dynamic/landgear/Simple/left/纵向摩擦力 ==
  note: 滚动摩擦系数
  note: 刹车摩擦系数，采用轮胎的魔术公式
      | μ = D sin(C*atan(Bλ))
      | 其中λ是滑移率
  BusElementIn3 : Inport  PortName=gear  Element=lambda
  BusElementIn2 : Inport  PortName=gear  Element=istatic
  BusElementIn4 : Inport  PortName=gear  Element=reaction
  BusElementIn1 : Inport  PortName=gear  Element=speed
  |Fz| : Inport  Port=2
  B : Gain  Gain=14.032
  C : Gain  Gain=1.5344
  Constant : Constant  Value=0.02
  D : Gain  Gain=0.8
  Product : Product
  Product1 : Product
  Selector : Selector  InputPortWidth=3  IndexOptions=Index vector (dialog)  Indices=1  OutputSizes=1
  Selector1 : Selector  InputPortWidth=2  IndexOptions=Index vector (dialog)  Indices=1  OutputSizes=1
  Selector5 : Selector  InputPortWidth=3  IndexOptions=Index vector (dialog)  Indices=1  OutputSizes=1
  Sign : Signum
  Sin : Trigonometry
  Sin1 : Trigonometry  Operator=atan
  Sum : Sum  Inputs=|++
  Switch : Switch  Criteria=u2 > Threshold  Threshold=0.5  SaturateOnIntegerOverflow=off  InputSameDT=off
  Unary Minus : UnaryMinus
  Fx : Outport
  wires:
  Sum/1 -> Product/1
  Unary Minus/1 -> Switch/3
  |Fz|/1 -> Product/2
  Product/1 -> Unary Minus/1
  Product1/1 -> Sum/2
  Sign/1 -> Product1/2
  Selector/1 -> Sign/1
  BusElementIn1/1 -> Selector/1
  Selector1/1 -> Switch/2
  BusElementIn2/1 -> Selector1/1
  Selector5/1 -> Switch/1
  Switch/1 -> Fx/1
  BusElementIn4/1 -> Selector5/1
  D/1 -> Sum/1
  Constant/1 -> Product1/1
  C/1 -> Sin/1
  Sin1/1 -> C/1
  B/1 -> Sin1/1
  Sin/1 -> D/1
  BusElementIn3/1 -> B/1

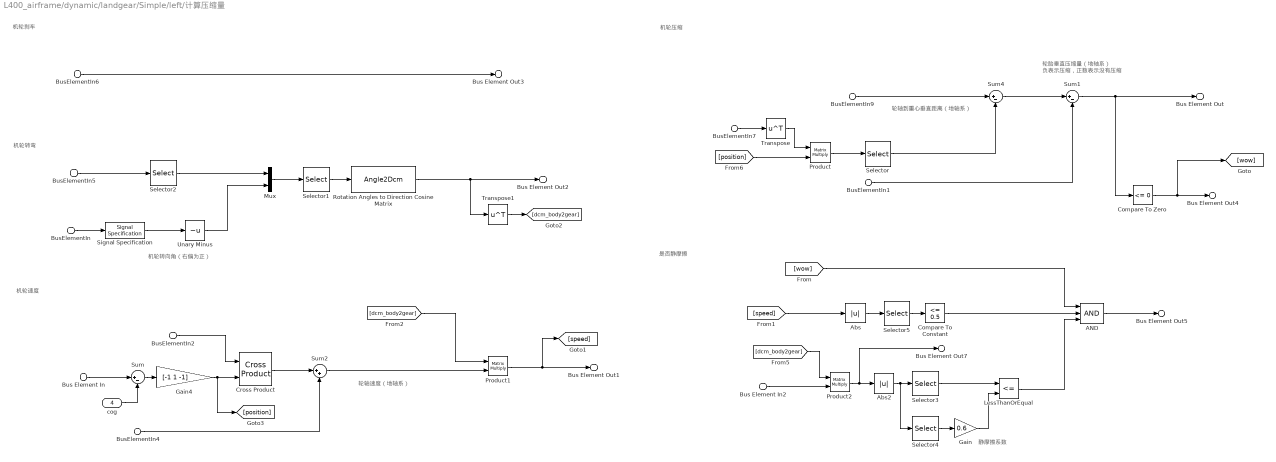
== system L400_airframe/dynamic/landgear/Simple/left/计算压缩量 ==
  note: 轮轴速度（地轴系）
  note: 轮轴到重心垂直距离（地轴系）
  note: 轮胎垂直压缩量（地轴系）
      | 负表示压缩，正数表示没有压缩
  note: 机轮转向角（右偏为正）
  note: 机轮压缩
  note: 机轮转弯
  note: 机轮速度
  note: 是否静摩擦
  note: 机轮刹车
  note: 静摩擦系数
  BusElementIn : Inport  PortName=cmd  Element=DWheel
  BusElementIn6 : Inport  PortName=cmd  Element=DBrake
  BusElementIn7 : Inport  Port=2  PortName=state  Element=aircraft.attitude.Rbe
  BusElementIn2 : Inport  Port=2  PortName=state  Element=aircraft.attitude.p_q_r
  BusElementIn5 : Inport  Port=2  PortName=state  Element=aircraft.attitude.phi_theta_psi
  BusElementIn4 : Inport  Port=2  PortName=state  Element=aircraft.position.vx_vy_vz
  BusElementIn9 : Inport  Port=2  PortName=state  Element=aircraft.position.alt
  BusElementIn1 : Inport  Port=2  PortName=state  Element=environ.terrain.hground
  Bus Element In : Inport  Port=3  PortName=param  Element=position
  Bus Element In2 : Inport  Port=3  PortName=param  Element=reaction
  cog : Inport  Port=4
  AND : Logic  Inputs=3  IconShape=distinctive  AllPortsSameDT=off  OutDataTypeStr=boolean
  Abs : Abs  SaturateOnIntegerOverflow=off
  Abs2 : Abs  SaturateOnIntegerOverflow=off
  Compare To Constant : simulink/Logic and Bit Operations/Compare To Constant  relop=<=  const=0.5  OutDataTypeStr=boolean
  Compare To Zero : simulink/Logic and Bit Operations/Compare To Zero  relop=<=  OutDataTypeStr=boolean
  Cross Product : matrix_library/Cross Product
  Gain : Gain  Gain=0.6
  Gain4 : Gain  Gain=[-1 1 -1]
  LessThanOrEqual : RelationalOperator  Operator=<=  OutDataTypeStr=boolean  RndMeth=Simplest  InputSameDT=off
  Mux : Mux  Inputs=2
  Product : Product  Multiplication=Matrix(*)
  Product1 : Product  Multiplication=Matrix(*)
  Product2 : Product  Multiplication=Matrix(*)
  Rotation Angles to Direction Cosine Matrix : Angle2Dcm
      settings: AttributesFormatString=Rotation Order: %<rotationOrder>
  Selector : Selector  InputPortWidth=3  IndexOptions=Index vector (dialog)  Indices=3  OutputSizes=1
  Selector1 : Selector  InputPortWidth=3  IndexOptions=Index vector (dialog)  Indices=[3 2 1]  OutputSizes=1
  Selector2 : Selector  InputPortWidth=3  IndexOptions=Index vector (dialog)  Indices=[1 2]  OutputSizes=1
  Selector3 : Selector  InputPortWidth=3  IndexOptions=Index vector (dialog)  Indices=[1 2]  OutputSizes=1
  Selector4 : Selector  InputPortWidth=3  IndexOptions=Index vector (dialog)  Indices=3  OutputSizes=1
  Selector5 : Selector  InputPortWidth=3  IndexOptions=Index vector (dialog)  Indices=[1 2]  OutputSizes=1
  Signal Specification : SignalSpecification  Unit=rad
  Sum : Sum  Inputs=|+-
  Sum1 : Sum  Inputs=|+-
  Sum2 : Sum  Inputs=|++
  Sum4 : Sum  Inputs=|+-
  Transpose : Math  Operator=transpose
  Transpose1 : Math  Operator=transpose
  Unary Minus : UnaryMinus
  Bus Element Out : Outport  PortName=gear  Element=cmprs
  Bus Element Out1 : Outport  PortName=gear  Element=speed
  Bus Element Out2 : Outport  PortName=gear  Element=dcm_gear2body
  Bus Element Out3 : Outport  PortName=gear  Element=lambda
  Bus Element Out4 : Outport  PortName=gear  Element=wow
  Bus Element Out5 : Outport  PortName=gear  Element=istatic
  Bus Element Out7 : Outport  PortName=gear  Element=reaction
  wires:
  Selector3/1 -> LessThanOrEqual/1
  Abs2/1 -> Selector3/1, Selector4/1
  Unary Minus/1 -> Mux/2
  Selector2/1 -> Mux/1
  BusElementIn5/1 -> Selector2/1
  Gain4/1 -> Cross Product/2, [position]
  Sum/1 -> Gain4/1
  cog/1 -> Sum/2
  Bus Element In/1 -> Sum/1
  AND/1 -> Bus Element Out5/1
  LessThanOrEqual/1 -> AND/3
  Gain/1 -> LessThanOrEqual/2
  Selector4/1 -> Gain/1
  Product2/1 -> Bus Element Out7/1, Abs2/1
  [dcm_body2gear] -> Product2/1
  Transpose1/1 -> [dcm_body2gear]
  [speed] -> Abs/1
  [wow] -> AND/1
  Abs/1 -> Selector5/1
  Compare To Constant/1 -> AND/2
  [dcm_body2gear] -> Product1/1
  Bus Element In2/1 -> Product2/2
  Rotation Angles to Direction Cosine Matrix/1 -> Transpose1/1, Bus Element Out2/1
  Selector1/1 -> Rotation Angles to Direction Cosine Matrix/1
  BusElementIn6/1 -> Bus Element Out3/1
  BusElementIn2/1 -> Cross Product/1
  BusElementIn1/1 -> Sum1/2
  Cross Product/1 -> Sum2/1
  Sum1/1 -> Bus Element Out/1, Compare To Zero/1
  BusElementIn4/1 -> Sum2/2
  [position] -> Product/2
  Transpose/1 -> Product/1
  Selector/1 -> Sum4/2
  BusElementIn9/1 -> Sum4/1
  Product/1 -> Selector/1
  Sum2/1 -> Product1/2
  Sum4/1 -> Sum1/1
  BusElementIn7/1 -> Transpose/1
  Compare To Zero/1 -> Bus Element Out4/1, [wow]
  Product1/1 -> Bus Element Out1/1, [speed]
  Mux/1 -> Selector1/1
  Signal Specification/1 -> Unary Minus/1
  BusElementIn/1 -> Signal Specification/1
  Selector5/1 -> Compare To Constant/1

== system L400_airframe/dynamic/landgear/Simple/rear/侧向摩擦力 ==
  note: % Compute the sideforce coefficients using Pacejka's Magic Formula.
      | %
      | % y(x) = D sin {C arctan [Bx - E(Bx - arctan Bx)]}
      | %
      | % Where: B = Stiffness Factor (0.06, here)
      | % C = Shape Factor (2.8, here)
      | % D = Peak Factor (0.8, here)
      | % E = Curvature Factor (1.03, here)
  Bus Element In3 : Inport  PortName=gear  Element=speed
  Bus Element In2 : Inport  PortName=gear  Element=istatic
  Bus Element In1 : Inport  PortName=gear  Element=reaction
  |Fz| : Inport  Port=2
  Angle Conversion : aerolibconvert2/Angle Conversion  IU=rad  OU=deg
  Atan : Trigonometry  Operator=atan
  Atan1 : Trigonometry  Operator=atan
  Atan2 : Trigonometry  Operator=atan2
  Atan3 : Trigonometry
  Demux : Demux  Outputs=2
  Gain : Gain  Gain=0.06
  Gain1 : Gain  Gain=1.03
  Gain2 : Gain  Gain=2.8
  Gain3 : Gain  Gain=0.8
  Product : Product
  Selector1 : Selector  InputPortWidth=3  IndexOptions=Index vector (dialog)  Indices=[2, 1]  OutputSizes=1
  Selector2 : Selector  InputPortWidth=2  IndexOptions=Index vector (dialog)  Indices=2  OutputSizes=1
  Selector3 : Selector  InputPortWidth=3  IndexOptions=Index vector (dialog)  Indices=2  OutputSizes=1
  Sum : Sum  Inputs=+-|
  Sum1 : Sum  Inputs=|+-
  Switch : Switch  Criteria=u2 > Threshold  Threshold=0.5  SaturateOnIntegerOverflow=off  InputSameDT=off
  Unary Minus : UnaryMinus
  Fy : Outport
  wires:
  Switch/1 -> Fy/1
  Bus Element In3/1 -> Selector1/1
  Demux/2 -> Atan2/2
  Selector1/1 -> Demux/1
  Demux/1 -> Atan2/1
  Selector2/1 -> Switch/2
  Bus Element In2/1 -> Selector2/1
  Bus Element In1/1 -> Selector3/1
  Selector3/1 -> Switch/1
  Product/1 -> Unary Minus/1
  Gain/1 -> Sum/1, Sum1/1, Atan/1
  Atan/1 -> Sum/2
  Gain2/1 -> Atan3/1
  Sum1/1 -> Atan1/1
  Sum/1 -> Gain1/1
  Atan1/1 -> Gain2/1
  Gain1/1 -> Sum1/2
  Atan2/1 -> Angle Conversion/1
  Atan3/1 -> Gain3/1
  Angle Conversion/1 -> Gain/1
  Gain3/1 -> Product/1
  |Fz|/1 -> Product/2
  Unary Minus/1 -> Switch/3

== system L400_airframe/dynamic/landgear/Simple/rear/地面支反力 ==
  note: 阻尼力
  note: 起落架缓冲器所提供的缓冲力是起落架提供给飞机支反力的主要组成部分，主要由随压缩行程变化的弹簧力、随压缩速率变化的阻尼力以及缓冲器内部有相对运动而产生的滑动摩擦力组成。
  note: 弹簧力
  note: 摩擦力
  note: 轮胎支反力
  note: 弹簧力刚度系数可以大概如下估算：
      | 无人机重力8000N，一共3个轮胎，假设平衡时轮胎压缩1cm，那么
      | K = 8000/3/0.01 ≈ 2.5e5
      | 弹簧系数一定不要打了，否则很容易发散
  Bus Element In1 : Inport  PortName=gear  Element=cmprs
  Bus Element In2 : Inport  PortName=gear  Element=speed
  Gain2 : Gain  Gain=1e5
  Gain3 : Gain  Gain=-1e3
  Gain7 : Gain  Gain=0
  Saturation : Saturate  UpperLimit=0  LowerLimit=-1
  Selector3 : Selector  InputPortWidth=3  IndexOptions=Index vector (dialog)  Indices=3  OutputSizes=1
  Sign : Signum
  Sum3 : Sum  Inputs=3
  Fz : Outport
  wires:
  Gain7/1 -> Sum3/3
  Bus Element In2/1 -> Selector3/1
  Sum3/1 -> Fz/1
  Sign/1 -> Gain7/1
  Saturation/1 -> Gain2/1
  Selector3/1 -> Sign/1, Gain3/1
  Gain3/1 -> Sum3/2
  Gain2/1 -> Sum3/1
  Bus Element In1/1 -> Saturation/1

== system L400_airframe/dynamic/landgear/Simple/rear/纵向摩擦力 ==
  note: 刹车摩擦系数，采用轮胎的魔术公式
      | μ = D sin(C*atan(Bλ))
      | 其中λ是滑移率
  note: 滚动摩擦系数
  BusElementIn3 : Inport  PortName=gear  Element=lambda
  BusElementIn2 : Inport  PortName=gear  Element=istatic
  BusElementIn4 : Inport  PortName=gear  Element=reaction
  BusElementIn1 : Inport  PortName=gear  Element=speed
  |Fz| : Inport  Port=2
  B : Gain  Gain=14.032
  C : Gain  Gain=1.5344
  Constant : Constant  Value=0.02
  D : Gain  Gain=0.8
  Product : Product
  Product1 : Product
  Selector : Selector  InputPortWidth=3  IndexOptions=Index vector (dialog)  Indices=1  OutputSizes=1
  Selector1 : Selector  InputPortWidth=2  IndexOptions=Index vector (dialog)  Indices=1  OutputSizes=1
  Selector5 : Selector  InputPortWidth=3  IndexOptions=Index vector (dialog)  Indices=1  OutputSizes=1
  Sign : Signum
  Sin : Trigonometry
  Sin1 : Trigonometry  Operator=atan
  Sum : Sum  Inputs=|++
  Switch : Switch  Criteria=u2 > Threshold  Threshold=0.5  SaturateOnIntegerOverflow=off  InputSameDT=off
  Unary Minus : UnaryMinus
  Fx : Outport
  wires:
  BusElementIn3/1 -> B/1
  Sin/1 -> D/1
  B/1 -> Sin1/1
  Sin1/1 -> C/1
  C/1 -> Sin/1
  Constant/1 -> Product1/1
  D/1 -> Sum/1
  BusElementIn4/1 -> Selector5/1
  Switch/1 -> Fx/1
  Selector5/1 -> Switch/1
  BusElementIn2/1 -> Selector1/1
  Selector1/1 -> Switch/2
  BusElementIn1/1 -> Selector/1
  Selector/1 -> Sign/1
  Sign/1 -> Product1/2
  Product1/1 -> Sum/2
  Product/1 -> Unary Minus/1
  |Fz|/1 -> Product/2
  Unary Minus/1 -> Switch/3
  Sum/1 -> Product/1
